simulink model "test_phase_voltages_without_delays"  (R2022a)
settings: Solver=FixedStepDiscrete  StartTime=0.0  StopTime=10.0  RelTol=1e-3
undefined symbols (not defined in the file or in its folder): f_c, Rt, u_dc
libraries: hdlsllib x3, simulink x2
(part 1 of 2)
settings Model: DataTypeOverride=Off  Creator=Andre Merx  LastModifiedBy=Andre Merx
settings SolverCC: AlgebraicLoopSolver=TrustRegion
settings DataIOCC: LimitDataPoints=on  SaveOutput=off  SaveTime=off
settings OptimizationCC: BlockReduction=off  ConditionallyExecuteInputs=off  DefaultParameterBehavior=Inlined  LifeSpan=inf
settings DebuggingCC: AlgebraicLoopMsg=error  SingleTaskRateTransMsg=error  UnconnectedInputMsg=warning  UnconnectedOutputMsg=warning  UnconnectedLineMsg=warning  AllowSymbolicDim=off  StrictBusMsg=ErrorOnBusTreatedAsVector  SFUnexpectedBacktrackingDiag=warning  SFNoUnconditionalDefaultTransitionDiag=warning  SFExecutionAtInitializationDiag=none  SFMachineParentedDataDiag=warning  ArithmeticOperatorsInVariantConditions=warning
settings HardwareCC: ProdBitPerPointer=32  ProdBitPerSizeT=32  ProdBitPerPtrDiffT=32  ProdLargestAtomicFloat=None  ProdIntDivRoundTo=Undefined  ProdEndianess=Unspecified  ProdWordSize=32  ProdHWDeviceType=ASIC/FPGA->ASIC/FPGA  ProdEqTarget=off
settings SFSimCC: SimUseLocalCustomCode=off  CustomCodeUndefinedFunction=UseInterfaceOnly
settings RTWCC: RTWUseLocalCustomCode=off
settings CodeAppCC: StateflowObjectComments=on
settings GRTTargetCC: TargetLangStandard=C89/C90 (ANSI)
settings ConfigComp: CovScope=ReferencedModels  CovMetricSettings=dw  CovSaveCumulativeToWorkspaceVar=on  CovSaveSingleToWorkspaceVar=on  CovExternalEMLEnable=off  CovSFcnEnable=off

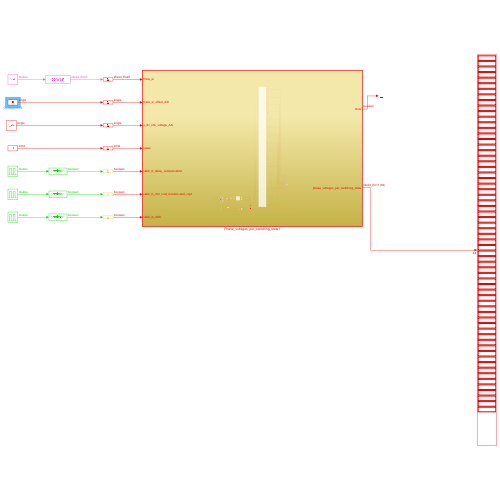
[thumbnail: Simulink's stored preview of the top-level diagram]
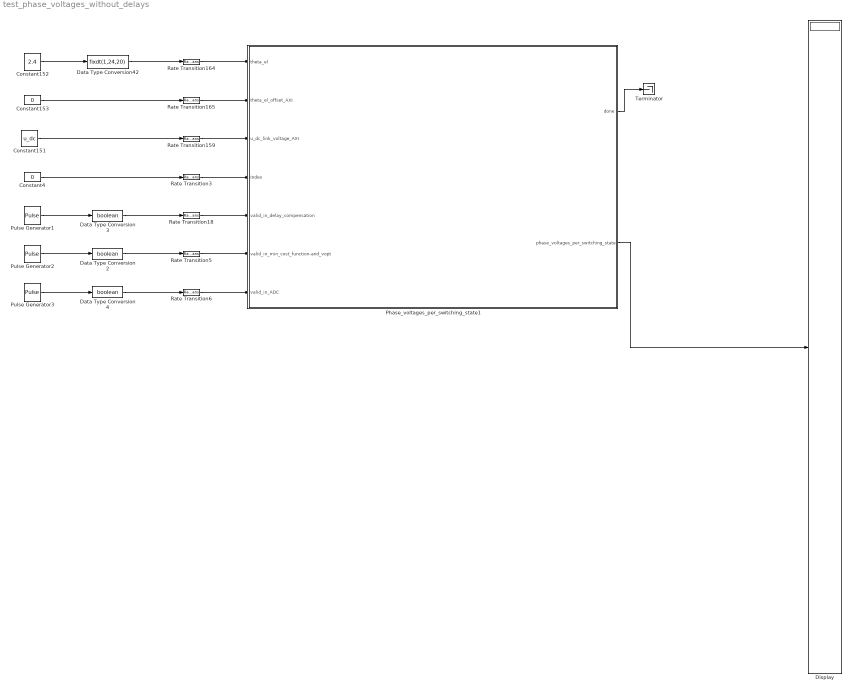
== system test_phase_voltages_without_delays ==
  Constant151 : Constant  Value=u_dc  OutDataTypeStr=single  SampleTime=-1
  Constant152 : Constant  Value=2.4
  Constant153 : Constant  Value=0  OutDataTypeStr=fixdt(1,24,20)  SampleTime=-1
  Constant4 : Constant  Value=0  OutDataTypeStr=int32  SampleTime=-1
  Data Type Conversion2 : DataTypeConversion  OutDataTypeStr=boolean  SaturateOnIntegerOverflow=off  RndMeth=Floor
  Data Type Conversion3 : DataTypeConversion  OutDataTypeStr=boolean  SaturateOnIntegerOverflow=off  RndMeth=Floor
  Data Type Conversion4 : DataTypeConversion  OutDataTypeStr=boolean  SaturateOnIntegerOverflow=off  RndMeth=Floor
  Data Type Conversion42 : DataTypeConversion  OutDataTypeStr=fixdt(1,24,20)  SaturateOnIntegerOverflow=off  RndMeth=Floor
  Display : Display
  Phase_voltages_per_switching_state1 : Subsystem  TreatAsAtomicUnit=on
  Pulse Generator1 : DiscretePulseGenerator  PulseType=Time based  Period=1/f_c
  Pulse Generator2 : DiscretePulseGenerator  PulseType=Time based  Period=1/f_c
  Pulse Generator3 : DiscretePulseGenerator  PulseType=Time based  Period=1/f_c
  Rate Transition{3,5..6,18,159,164..165} (7 alike) : RateTransition  OutPortSampleTime=Rt
  Terminator : Terminator
  wires:
  Rate Transition165/1 -> Phase_voltages_per_switching_state1/2(theta_el_offset_AXI)
  Rate Transition164/1 -> Phase_voltages_per_switching_state1/1(theta_el)
  Rate Transition159/1 -> Phase_voltages_per_switching_state1/3(u_dc_link_voltage_AXI)
  Constant152/1 -> Data Type Conversion42/1
  Constant153/1 -> Rate Transition165/1
  Constant151/1 -> Rate Transition159/1
  Data Type Conversion42/1 -> Rate Transition164/1
  Data Type Conversion3/1 -> Rate Transition18/1
  Rate Transition6/1 -> Phase_voltages_per_switching_state1/7(valid_in_ADC)
  Rate Transition18/1 -> Phase_voltages_per_switching_state1/5(valid_in_delay_compensation)
  Pulse Generator1/1 -> Data Type Conversion3/1
  Rate Transition3/1 -> Phase_voltages_per_switching_state1/4(Index)
  Data Type Conversion4/1 -> Rate Transition6/1
  Constant4/1 -> Rate Transition3/1
  Data Type Conversion2/1 -> Rate Transition5/1
  Pulse Generator3/1 -> Data Type Conversion4/1
  Rate Transition5/1 -> Phase_voltages_per_switching_state1/6(valid_in_min_cost_function-and_vopt)
  Pulse Generator2/1 -> Data Type Conversion2/1
  Phase_voltages_per_switching_state1/1(done) -> Terminator/1
  Phase_voltages_per_switching_state1/2(phase_voltages_per_switching_state) -> Display/1

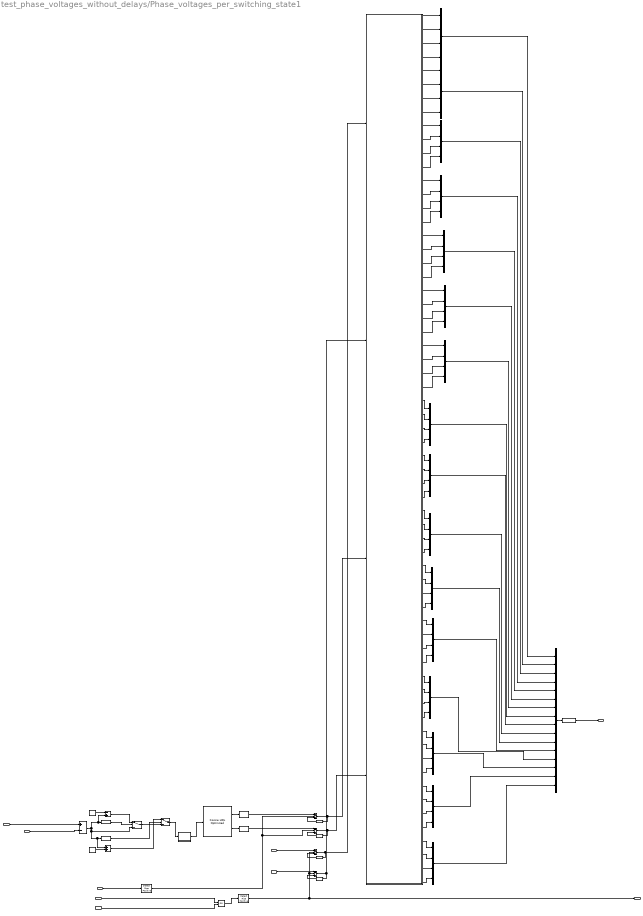
== system test_phase_voltages_without_delays/Phase_voltages_per_switching_state1 ==
  theta_el : Inport
  theta_el_offset_AXI : Inport  Port=2
  u_dc_link_voltage_AXI : Inport  Port=3
  Index : Inport  Port=4
  valid_in_delay_compensation : Inport  Port=5
  valid_in_min_cost_function-and_vopt : Inport  Port=6
  valid_in_ADC : Inport  Port=7
  Add1 : Sum  Inputs=+-  OutDataTypeStr=fixdt(1,24,20)
  Add2 : Sum  Inputs=-+  OutDataTypeStr=fixdt(1,24,20)
  Add3 : Sum  OutDataTypeStr=fixdt(1,24,20)
  Compare Limit_High : simulink/Logic and Bit Operations/Compare To Constant  relop=>=  const=2*pi  OutDataTypeStr=boolean
  Compare Limit_Low : simulink/Logic and Bit Operations/Compare To Constant  relop=<  const=0  OutDataTypeStr=boolean
  Constant : Constant  Value=2*pi  OutDataTypeStr=fixdt(1,24,20)  SampleTime=Rt
  Constant1 : Constant  Value=2*pi  OutDataTypeStr=fixdt(1,24,20)  SampleTime=Rt
  Data Type Conversion1 : DataTypeConversion  OutDataTypeStr=fixdt(1,24,11)  SaturateOnIntegerOverflow=off  RndMeth=Floor
  Data Type Conversion2 : DataTypeConversion  OutDataTypeStr=single  SaturateOnIntegerOverflow=off  RndMeth=Floor
  Data Type Conversion42 : DataTypeConversion  OutDataTypeStr=single  SaturateOnIntegerOverflow=off  RndMeth=Floor
  Delay{1..2,13..14} (4 alike) : Delay  DelayLength=1
  Detect Rise Positive : hdlsllib/Logic and Bit Operations/Detect Rise Positive  vinit=0  OutDataTypeStr=boolean
      settings: SourceProductBaseCode=SL
  Detect Rise Positive1 : hdlsllib/Logic and Bit Operations/Detect Rise Positive  vinit=0  OutDataTypeStr=boolean
      settings: SourceProductBaseCode=SL
  Logical Operator : Logic  Operator=OR  AllPortsSameDT=off  OutDataTypeStr=boolean
  MATLAB Function1 : MATLAB Function  TreatAsAtomicUnit=on
  Mux{,1..15} (16 alike) : Mux
  Mux16 : Mux  Inputs=16
  Sine HDL Optimized : hdlsllib/Lookup Tables/Cosine HDL Optimized  OutputFormula=sin(2*pi*u) and cos(2*pi*u)  NumDataPoints=64  TableDataTypeStr=fixdt(1,24,20)  SimulateLUTROMDelay=off
      settings: SourceProductBaseCode=SL
  Subsystem : Subsystem
  Switch_Limit_High : Switch  Criteria=u2 > Threshold  OutDataTypeStr=fixdt(1,24,20)  SaturateOnIntegerOverflow=off  InputSameDT=off
  Switch_Limit_Low : Switch  Criteria=u2 > Threshold  OutDataTypeStr=fixdt(1,24,20)  SaturateOnIntegerOverflow=off  InputSameDT=off
  Switch_on1 : Switch  Threshold=1  OutDataTypeStr=single  RndMeth=Simplest  SaturateOnIntegerOverflow=off  InputSameDT=off
  Switch_on13 : Switch  Threshold=1  OutDataTypeStr=single  RndMeth=Simplest  SaturateOnIntegerOverflow=off  InputSameDT=off
  Switch_on2 : Switch  Threshold=1  OutDataTypeStr=single  RndMeth=Simplest  SaturateOnIntegerOverflow=off  InputSameDT=off
  Switch_on3 : Switch  Threshold=1  OutDataTypeStr=int32  RndMeth=Simplest  SaturateOnIntegerOverflow=off  InputSameDT=off
  done : Outport
  phase_voltages_per_switching_state : Outport  Port=2
  wires:
  Compare Limit_High/1 -> Switch_Limit_High/2
  Delay14/1 -> Switch_on3/3
  Delay13/1 -> Switch_on13/3
  Switch_on13/1 -> Subsystem/4(cos_theta_el1), Delay13/1
  u_dc_link_voltage_AXI/1 -> Switch_on1/1  "End_Cycle"
  Switch_Limit_High/1 -> Switch_Limit_Low/3
  Constant/1 -> Add2/1
  theta_el_offset_AXI/1 -> Add1/2
  Add3/1 -> Switch_Limit_Low/1
  theta_el/1 -> Add1/1  "End_Cycle"
  Switch_Limit_Low/1 -> MATLAB Function1/1(u)  "End_Cycle"
  Add1/1 -> Switch_Limit_High/3, Add3/1, Compare Limit_Low/1, Add2/2, Compare Limit_High/1
  Switch_on1/1 -> Subsystem/1(u_dc_link_voltage15), Delay1/1
  Detect Rise Positive1/1 -> done/1, Switch_on3/2, Switch_on1/2  "End_Cycle"
  Compare Limit_Low/1 -> Switch_Limit_Low/2
  Delay1/1 -> Switch_on1/3
  Constant1/1 -> Add3/2
  Add2/1 -> Switch_Limit_High/1
  Index/1 -> Switch_on3/1  "End_Cycle"
  Logical Operator/1 -> Detect Rise Positive1/1
  Switch_on3/1 -> Delay14/1, Subsystem/2(Index 15)
  Subsystem/61(d_voltage_per_switching_state15) -> Mux/1
  Subsystem/62(q_voltage_per_switching_state15) -> Mux/2
  Subsystem/63(x_voltage_per_switching_state15) -> Mux/3
  Subsystem/64(y_voltage_per_switching_state15) -> Mux/4
  Subsystem/1(d_voltage_per_switching_state) -> Mux1/1
  Subsystem/2(q_voltage_per_switching_state) -> Mux1/2
  Subsystem/4(y_voltage_per_switching_state) -> Mux1/4
  Subsystem/3(x_voltage_per_switching_state) -> Mux1/3
  Subsystem/7(x_voltage_per_switching_state1) -> Mux2/3
  Subsystem/5(d_voltage_per_switching_state1) -> Mux2/1
  Subsystem/6(q_voltage_per_switching_state1) -> Mux2/2
  Subsystem/8(y_voltage_per_switching_state1) -> Mux2/4
  Subsystem/12(y_voltage_per_switching_state2) -> Mux3/4
  Subsystem/9(d_voltage_per_switching_state2) -> Mux3/1
  Subsystem/10(q_voltage_per_switching_state2) -> Mux3/2
  Subsystem/11(x_voltage_per_switching_state2) -> Mux3/3
  Subsystem/13(d_voltage_per_switching_state3) -> Mux4/1
  Subsystem/15(x_voltage_per_switching_state3) -> Mux4/3
  Subsystem/16(y_voltage_per_switching_state3) -> Mux4/4
  Subsystem/14(q_voltage_per_switching_state3) -> Mux4/2
  Subsystem/19(x_voltage_per_switching_state4) -> Mux5/3
  Subsystem/18(q_voltage_per_switching_state4) -> Mux5/2
  Subsystem/17(d_voltage_per_switching_state4) -> Mux5/1
  Subsystem/20(y_voltage_per_switching_state4) -> Mux5/4
  Subsystem/23(x_voltage_per_switching_state5) -> Mux6/3
  Subsystem/21(d_voltage_per_switching_state5) -> Mux6/1
  Subsystem/22(q_voltage_per_switching_state5) -> Mux6/2
  Subsystem/24(y_voltage_per_switching_state5) -> Mux6/4
  Subsystem/25(d_voltage_per_switching_state6) -> Mux7/1
  Subsystem/28(y_voltage_per_switching_state6) -> Mux7/4
  Subsystem/27(x_voltage_per_switching_state6) -> Mux7/3
  Subsystem/26(q_voltage_per_switching_state6) -> Mux7/2
  Subsystem/29(d_voltage_per_switching_state7) -> Mux8/1
  Subsystem/32(y_voltage_per_switching_state7) -> Mux8/4
  Subsystem/30(q_voltage_per_switching_state7) -> Mux8/2
  Subsystem/31(x_voltage_per_switching_state7) -> Mux8/3
  Subsystem/36(y_voltage_per_switching_state8) -> Mux9/4
  Subsystem/33(d_voltage_per_switching_state8) -> Mux9/1
  Subsystem/34(q_voltage_per_switching_state8) -> Mux9/2
  Subsystem/35(x_voltage_per_switching_state8) -> Mux9/3
  Mux10/1 -> Mux16/10
  Subsystem/40(y_voltage_per_switching_state9) -> Mux10/4
  Subsystem/39(x_voltage_per_switching_state9) -> Mux10/3
  Subsystem/37(d_voltage_per_switching_state9) -> Mux10/1
  Subsystem/38(q_voltage_per_switching_state9) -> Mux10/2
  Subsystem/43(x_voltage_per_switching_state10) -> Mux11/3
  Subsystem/41(d_voltage_per_switching_state10) -> Mux11/1
  Subsystem/42(q_voltage_per_switching_state10) -> Mux11/2
  Subsystem/44(y_voltage_per_switching_state10) -> Mux11/4
  Mux12/1 -> Mux16/12
  Subsystem/48(y_voltage_per_switching_state11) -> Mux12/4
  Subsystem/46(q_voltage_per_switching_state11) -> Mux12/2
  Subsystem/47(x_voltage_per_switching_state11) -> Mux12/3
  Subsystem/45(d_voltage_per_switching_state11) -> Mux12/1
  Subsystem/52(y_voltage_per_switching_state12) -> Mux13/4
  Subsystem/50(q_voltage_per_switching_state12) -> Mux13/2
  Subsystem/51(x_voltage_per_switching_state12) -> Mux13/3
  Subsystem/49(d_voltage_per_switching_state12) -> Mux13/1
  Mux14/1 -> Mux16/14
  Subsystem/56(y_voltage_per_switching_state13) -> Mux14/4
  Subsystem/53(d_voltage_per_switching_state13) -> Mux14/1
  Subsystem/55(x_voltage_per_switching_state13) -> Mux14/3
  Subsystem/54(q_voltage_per_switching_state13) -> Mux14/2
  Subsystem/57(d_voltage_per_switching_state14) -> Mux15/1
  Subsystem/60(y_voltage_per_switching_state14) -> Mux15/4
  Subsystem/59(x_voltage_per_switching_state14) -> Mux15/3
  Subsystem/58(q_voltage_per_switching_state14) -> Mux15/2
  Mux15/1 -> Mux16/15
  Mux16/1 -> Data Type Conversion1/1
  Mux1/1 -> Mux16/1
  Mux2/1 -> Mux16/2
  Mux3/1 -> Mux16/3
  Mux4/1 -> Mux16/4
  Mux5/1 -> Mux16/5
  Mux6/1 -> Mux16/6
  Mux7/1 -> Mux16/7
  Mux8/1 -> Mux16/8
  Mux9/1 -> Mux16/9
  Mux11/1 -> Mux16/11
  Mux13/1 -> Mux16/13
  Mux/1 -> Mux16/16
  Data Type Conversion1/1 -> phase_voltages_per_switching_state/1
  valid_in_ADC/1 -> Detect Rise Positive/1
  valid_in_delay_compensation/1 -> Logical Operator/1
  valid_in_min_cost_function-and_vopt/1 -> Logical Operator/2
  MATLAB Function1/1(y) -> Sine HDL Optimized/1
  Sine HDL Optimized/1 -> Data Type Conversion42/1
  Detect Rise Positive/1 -> Switch_on13/2, Switch_on2/2  "End_Cycle"
  Delay2/1 -> Switch_on2/3
  Switch_on2/1 -> Subsystem/3(sin_theta_el), Delay2/1
  Sine HDL Optimized/2 -> Data Type Conversion2/1
  Data Type Conversion42/1 -> Switch_on2/1
  Data Type Conversion2/1 -> Switch_on13/1

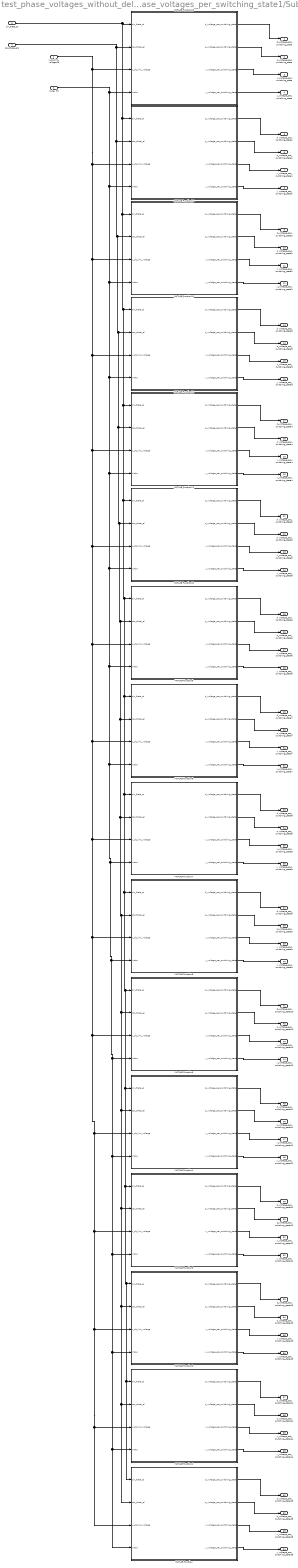
== system test_phase_voltages_without_delays/Phase_voltages_per_switching_state1/Subsystem ==
  u_dc_link_voltage15 : Inport
  Index 15 : Inport  Port=2
  sin_theta_el : Inport  Port=3
  cos_theta_el1 : Inport  Port=4
  MATLAB Function : MATLAB Function  TreatAsAtomicUnit=on
  MATLAB Function1 : MATLAB Function  TreatAsAtomicUnit=on
  MATLAB Function10 : MATLAB Function  TreatAsAtomicUnit=on
  MATLAB Function11 : MATLAB Function  TreatAsAtomicUnit=on
  MATLAB Function12 : MATLAB Function  TreatAsAtomicUnit=on
  MATLAB Function13 : MATLAB Function  TreatAsAtomicUnit=on
  MATLAB Function14 : MATLAB Function  TreatAsAtomicUnit=on
  MATLAB Function15 : MATLAB Function  TreatAsAtomicUnit=on
  MATLAB Function2 : MATLAB Function  TreatAsAtomicUnit=on
  MATLAB Function3 : MATLAB Function  TreatAsAtomicUnit=on
  MATLAB Function4 : MATLAB Function  TreatAsAtomicUnit=on
  MATLAB Function5 : MATLAB Function  TreatAsAtomicUnit=on
  MATLAB Function6 : MATLAB Function  TreatAsAtomicUnit=on
  MATLAB Function7 : MATLAB Function  TreatAsAtomicUnit=on
  MATLAB Function8 : MATLAB Function  TreatAsAtomicUnit=on
  MATLAB Function9 : MATLAB Function  TreatAsAtomicUnit=on
  d_voltage_per_switching_state : Outport
  q_voltage_per_switching_state : Outport  Port=2
  x_voltage_per_switching_state : Outport  Port=3
  y_voltage_per_switching_state : Outport  Port=4
  d_voltage_per_switching_state1 : Outport  Port=5
  q_voltage_per_switching_state1 : Outport  Port=6
  x_voltage_per_switching_state1 : Outport  Port=7
  y_voltage_per_switching_state1 : Outport  Port=8
  d_voltage_per_switching_state2 : Outport  Port=9
  q_voltage_per_switching_state2 : Outport  Port=10
  x_voltage_per_switching_state2 : Outport  Port=11
  y_voltage_per_switching_state2 : Outport  Port=12
  d_voltage_per_switching_state3 : Outport  Port=13
  q_voltage_per_switching_state3 : Outport  Port=14
  x_voltage_per_switching_state3 : Outport  Port=15
  y_voltage_per_switching_state3 : Outport  Port=16
  d_voltage_per_switching_state4 : Outport  Port=17
  q_voltage_per_switching_state4 : Outport  Port=18
  x_voltage_per_switching_state4 : Outport  Port=19
  y_voltage_per_switching_state4 : Outport  Port=20
  d_voltage_per_switching_state5 : Outport  Port=21
  q_voltage_per_switching_state5 : Outport  Port=22
  x_voltage_per_switching_state5 : Outport  Port=23
  y_voltage_per_switching_state5 : Outport  Port=24
  d_voltage_per_switching_state6 : Outport  Port=25
  q_voltage_per_switching_state6 : Outport  Port=26
  x_voltage_per_switching_state6 : Outport  Port=27
  y_voltage_per_switching_state6 : Outport  Port=28
  d_voltage_per_switching_state7 : Outport  Port=29
  q_voltage_per_switching_state7 : Outport  Port=30
  x_voltage_per_switching_state7 : Outport  Port=31
  y_voltage_per_switching_state7 : Outport  Port=32
  d_voltage_per_switching_state8 : Outport  Port=33
  q_voltage_per_switching_state8 : Outport  Port=34
  x_voltage_per_switching_state8 : Outport  Port=35
  y_voltage_per_switching_state8 : Outport  Port=36
  d_voltage_per_switching_state9 : Outport  Port=37
  q_voltage_per_switching_state9 : Outport  Port=38
  x_voltage_per_switching_state9 : Outport  Port=39
  y_voltage_per_switching_state9 : Outport  Port=40
  d_voltage_per_switching_state10 : Outport  Port=41
  q_voltage_per_switching_state10 : Outport  Port=42
  x_voltage_per_switching_state10 : Outport  Port=43
  y_voltage_per_switching_state10 : Outport  Port=44
  d_voltage_per_switching_state11 : Outport  Port=45
  q_voltage_per_switching_state11 : Outport  Port=46
  x_voltage_per_switching_state11 : Outport  Port=47
  y_voltage_per_switching_state11 : Outport  Port=48
  d_voltage_per_switching_state12 : Outport  Port=49
  q_voltage_per_switching_state12 : Outport  Port=50
  x_voltage_per_switching_state12 : Outport  Port=51
  y_voltage_per_switching_state12 : Outport  Port=52
  d_voltage_per_switching_state13 : Outport  Port=53
  q_voltage_per_switching_state13 : Outport  Port=54
  x_voltage_per_switching_state13 : Outport  Port=55
  y_voltage_per_switching_state13 : Outport  Port=56
  d_voltage_per_switching_state14 : Outport  Port=57
  q_voltage_per_switching_state14 : Outport  Port=58
  x_voltage_per_switching_state14 : Outport  Port=59
  y_voltage_per_switching_state14 : Outport  Port=60
  d_voltage_per_switching_state15 : Outport  Port=61
  q_voltage_per_switching_state15 : Outport  Port=62
  x_voltage_per_switching_state15 : Outport  Port=63
  y_voltage_per_switching_state15 : Outport  Port=64
  wires:
  MATLAB Function4/1(d_voltage_per_switching_state) -> d_voltage_per_switching_state11/1
  MATLAB Function11/4(y_voltage_per_switching_state) -> y_voltage_per_switching_state4/1
  MATLAB Function3/2(q_voltage_per_switching_state) -> q_voltage_per_switching_state12/1
  MATLAB Function3/4(y_voltage_per_switching_state) -> y_voltage_per_switching_state12/1
  MATLAB Function10/3(x_voltage_per_switching_state) -> x_voltage_per_switching_state5/1
  MATLAB Function8/1(d_voltage_per_switching_state) -> d_voltage_per_switching_state7/1
  MATLAB Function8/2(q_voltage_per_switching_state) -> q_voltage_per_switching_state7/1
  MATLAB Function3/1(d_voltage_per_switching_state) -> d_voltage_per_switching_state12/1
  MATLAB Function11/1(d_voltage_per_switching_state) -> d_voltage_per_switching_state4/1
  MATLAB Function12/3(x_voltage_per_switching_state) -> x_voltage_per_switching_state3/1
  MATLAB Function15/2(q_voltage_per_switching_state) -> q_voltage_per_switching_state/1
  MATLAB Function8/3(x_voltage_per_switching_state) -> x_voltage_per_switching_state7/1
  MATLAB Function/1(d_voltage_per_switching_state) -> d_voltage_per_switching_state15/1
  MATLAB Function11/3(x_voltage_per_switching_state) -> x_voltage_per_switching_state4/1
  MATLAB Function10/4(y_voltage_per_switching_state) -> y_voltage_per_switching_state5/1
  MATLAB Function4/3(x_voltage_per_switching_state) -> x_voltage_per_switching_state11/1
  MATLAB Function11/2(q_voltage_per_switching_state) -> q_voltage_per_switching_state4/1
  MATLAB Function12/1(d_voltage_per_switching_state) -> d_voltage_per_switching_state3/1
  MATLAB Function2/1(d_voltage_per_switching_state) -> d_voltage_per_switching_state13/1
  MATLAB Function12/4(y_voltage_per_switching_state) -> y_voltage_per_switching_state3/1
  MATLAB Function/3(x_voltage_per_switching_state) -> x_voltage_per_switching_state15/1
  MATLAB Function13/2(q_voltage_per_switching_state) -> q_voltage_per_switching_state2/1
  MATLAB Function10/1(d_voltage_per_switching_state) -> d_voltage_per_switching_state5/1
  MATLAB Function10/2(q_voltage_per_switching_state) -> q_voltage_per_switching_state5/1
  MATLAB Function4/4(y_voltage_per_switching_state) -> y_voltage_per_switching_state11/1
  MATLAB Function3/3(x_voltage_per_switching_state) -> x_voltage_per_switching_state12/1
  MATLAB Function13/4(y_voltage_per_switching_state) -> y_voltage_per_switching_state2/1
  MATLAB Function8/4(y_voltage_per_switching_state) -> y_voltage_per_switching_state7/1
  MATLAB Function13/1(d_voltage_per_switching_state) -> d_voltage_per_switching_state2/1
  MATLAB Function13/3(x_voltage_per_switching_state) -> x_voltage_per_switching_state2/1
  MATLAB Function1/4(y_voltage_per_switching_state) -> y_voltage_per_switching_state14/1
  MATLAB Function1/1(d_voltage_per_switching_state) -> d_voltage_per_switching_state14/1
  MATLAB Function12/2(q_voltage_per_switching_state) -> q_voltage_per_switching_state3/1
  MATLAB Function4/2(q_voltage_per_switching_state) -> q_voltage_per_switching_state11/1
  MATLAB Function6/2(q_voltage_per_switching_state) -> q_voltage_per_switching_state9/1
  MATLAB Function5/3(x_voltage_per_switching_state) -> x_voltage_per_switching_state10/1
  MATLAB Function6/3(x_voltage_per_switching_state) -> x_voltage_per_switching_state9/1
  MATLAB Function6/1(d_voltage_per_switching_state) -> d_voltage_per_switching_state9/1
  MATLAB Function6/4(y_voltage_per_switching_state) -> y_voltage_per_switching_state9/1
  MATLAB Function15/1(d_voltage_per_switching_state) -> d_voltage_per_switching_state/1
  MATLAB Function15/4(y_voltage_per_switching_state) -> y_voltage_per_switching_state/1
  MATLAB Function15/3(x_voltage_per_switching_state) -> x_voltage_per_switching_state/1
  MATLAB Function/4(y_voltage_per_switching_state) -> y_voltage_per_switching_state15/1
  MATLAB Function/2(q_voltage_per_switching_state) -> q_voltage_per_switching_state15/1
  u_dc_link_voltage15/1 -> MATLAB Function/3(u_dc_link_voltage), MATLAB Function1/3(u_dc_link_voltage), MATLAB Function2/3(u_dc_link_voltage), MATLAB Function3/3(u_dc_link_voltage), MATLAB Function4/3(u_dc_link_voltage), MATLAB Function5/3(u_dc_link_voltage), MATLAB Function6/3(u_dc_link_voltage), MATLAB Function7/3(u_dc_link_voltage), MATLAB Function8/3(u_dc_link_voltage), MATLAB Function9/3(u_dc_link_voltage), MATLAB Function10/3(u_dc_link_voltage), MATLAB Function11/3(u_dc_link_voltage), MATLAB Function12/3(u_dc_link_voltage), MATLAB Function13/3(u_dc_link_voltage), MATLAB Function14/3(u_dc_link_voltage), MATLAB Function15/3(u_dc_link_voltage)
  MATLAB Function14/4(y_voltage_per_switching_state) -> y_voltage_per_switching_state1/1
  MATLAB Function2/2(q_voltage_per_switching_state) -> q_voltage_per_switching_state13/1
  MATLAB Function14/3(x_voltage_per_switching_state) -> x_voltage_per_switching_state1/1
  MATLAB Function14/1(d_voltage_per_switching_state) -> d_voltage_per_switching_state1/1
  MATLAB Function14/2(q_voltage_per_switching_state) -> q_voltage_per_switching_state1/1
  Index 15/1 -> MATLAB Function15/4(Index), MATLAB Function10/4(Index), MATLAB Function8/4(Index), MATLAB Function/4(Index), MATLAB Function1/4(Index), MATLAB Function2/4(Index), MATLAB Function3/4(Index), MATLAB Function4/4(Index), MATLAB Function5/4(Index), MATLAB Function6/4(Index), MATLAB Function7/4(Index), MATLAB Function9/4(Index), MATLAB Function11/4(Index), MATLAB Function12/4(Index), MATLAB Function13/4(Index), MATLAB Function14/4(Index)
  MATLAB Function1/2(q_voltage_per_switching_state) -> q_voltage_per_switching_state14/1
  MATLAB Function1/3(x_voltage_per_switching_state) -> x_voltage_per_switching_state14/1
  MATLAB Function9/3(x_voltage_per_switching_state) -> x_voltage_per_switching_state6/1
  MATLAB Function9/2(q_voltage_per_switching_state) -> q_voltage_per_switching_state6/1
  MATLAB Function9/1(d_voltage_per_switching_state) -> d_voltage_per_switching_state6/1
  MATLAB Function9/4(y_voltage_per_switching_state) -> y_voltage_per_switching_state6/1
  MATLAB Function7/1(d_voltage_per_switching_state) -> d_voltage_per_switching_state8/1
  MATLAB Function7/4(y_voltage_per_switching_state) -> y_voltage_per_switching_state8/1
  MATLAB Function7/2(q_voltage_per_switching_state) -> q_voltage_per_switching_state8/1
  MATLAB Function7/3(x_voltage_per_switching_state) -> x_voltage_per_switching_state8/1
  MATLAB Function5/2(q_voltage_per_switching_state) -> q_voltage_per_switching_state10/1
  MATLAB Function5/1(d_voltage_per_switching_state) -> d_voltage_per_switching_state10/1
  MATLAB Function5/4(y_voltage_per_switching_state) -> y_voltage_per_switching_state10/1
  MATLAB Function2/3(x_voltage_per_switching_state) -> x_voltage_per_switching_state13/1
  MATLAB Function2/4(y_voltage_per_switching_state) -> y_voltage_per_switching_state13/1
  sin_theta_el/1 -> MATLAB Function14/1(sin_theta_el), MATLAB Function/1(sin_theta_el), MATLAB Function1/1(sin_theta_el), MATLAB Function2/1(sin_theta_el), MATLAB Function3/1(sin_theta_el), MATLAB Function4/1(sin_theta_el), MATLAB Function5/1(sin_theta_el), MATLAB Function6/1(sin_theta_el), MATLAB Function7/1(sin_theta_el), MATLAB Function8/1(sin_theta_el), MATLAB Function9/1(sin_theta_el), MATLAB Function10/1(sin_theta_el), MATLAB Function11/1(sin_theta_el), MATLAB Function12/1(sin_theta_el), MATLAB Function13/1(sin_theta_el), MATLAB Function15/1(sin_theta_el)
  cos_theta_el1/1 -> MATLAB Function15/2(cos_theta_el), MATLAB Function/2(cos_theta_el), MATLAB Function1/2(cos_theta_el), MATLAB Function2/2(cos_theta_el), MATLAB Function3/2(cos_theta_el), MATLAB Function4/2(cos_theta_el), MATLAB Function5/2(cos_theta_el), MATLAB Function6/2(cos_theta_el), MATLAB Function7/2(cos_theta_el), MATLAB Function8/2(cos_theta_el), MATLAB Function9/2(cos_theta_el), MATLAB Function10/2(cos_theta_el), MATLAB Function11/2(cos_theta_el), MATLAB Function12/2(cos_theta_el), MATLAB Function13/2(cos_theta_el), MATLAB Function14/2(cos_theta_el)

== matlab function test_phase_voltages_without_delays/Phase_voltages_per_switching_state1/Subsystem/MATLAB Function14 ==
  data: sin_theta_el input; cos_theta_el input; d_voltage_per_switching_state output; u_dc_link_voltage input; Index input; q_voltage_per_switching_state output; x_voltage_per_switching_state output; y_voltage_per_switching_state output
function [d_voltage_per_switching_state, q_voltage_per_switching_state, x_voltage_per_switching_state, y_voltage_per_switching_state] = fcn(sin_theta_el, cos_theta_el, u_dc_link_voltage, Index)
      
        % Initial condition
            Index = Index+1;

    
        % Swichtingstates factors alpha beta x y
        Factors_alpha_beta_x_y = single([-0.166666666666667	 0.166666666666667	-0.333333333333333	0;
                                         -0.288675134594813	-0.288675134594813	 0	                0;
                                         -0.166666666666667	 0.166666666666667	-0.333333333333333	0;
                                          0.288675134594813	 0.288675134594813	 0              	0]);
        
        % Park-Transformation of the switchingstates factors
        Factors_d_q_x_y =single(zeros(4,1));
    
        Factors_d_q_x_y(3,1) = Factors_alpha_beta_x_y(3,Index);
        Factors_d_q_x_y(4,1) = Factors_alpha_beta_x_y(4,Index);
       
        Factors_d_q_x_y(1,1) = cos_theta_el*Factors_alpha_beta_x_y(1,Index)+sin_theta_el*Factors_alpha_beta_x_y(2,Index);
        Factors_d_q_x_y(2,1) = -sin_theta_el*Factors_alpha_beta_x_y(1,Index)+cos_theta_el*Factors_alpha_beta_x_y(2,Index);
    
        %Calculation of the voltages per switching state in alpha beta coordinates
        d_q_x_y_voltages_per_switching_state = single(u_dc_link_voltage*Factors_d_q_x_y);
    
        d_voltage_per_switching_state = d_q_x_y_voltages_per_switching_state(1,1);
        q_voltage_per_switching_state = d_q_x_y_voltages_per_switching_state(2,1);
        x_voltage_per_switching_state = d_q_x_y_voltages_per_switching_state(3,1);
        y_voltage_per_switching_state = d_q_x_y_voltages_per_switching_state(4,1);
    

end

== matlab function test_phase_voltages_without_delays/Phase_voltages_per_switching_state1/Subsystem/MATLAB Function15 ==
  data: sin_theta_el input; cos_theta_el input; d_voltage_per_switching_state output; u_dc_link_voltage input; Index input; q_voltage_per_switching_state output; x_voltage_per_switching_state output; y_voltage_per_switching_state output
function [d_voltage_per_switching_state, q_voltage_per_switching_state, x_voltage_per_switching_state, y_voltage_per_switching_state] = fcn(sin_theta_el, cos_theta_el, u_dc_link_voltage, Index)
      
        % Initial condition
            Index = Index+1;

        % Swichtingstates factors alpha beta x y
        Factors_alpha_beta_x_y = single([0	    0.333333333333333	-0.166666666666667	 0.166666666666667;
                                         0	    0                    0.288675134594813	 0.288675134594813;
                                         0	    0.333333333333333	-0.166666666666667	 0.166666666666667;
                                         0	    0	                -0.288675134594813	-0.288675134594813]);
        
        % Park-Transformation of the switchingstates factors
        Factors_d_q_x_y =single(zeros(4,1));
    
        Factors_d_q_x_y(3,1) = Factors_alpha_beta_x_y(3,Index);
        Factors_d_q_x_y(4,1) = Factors_alpha_beta_x_y(4,Index);
          
        Factors_d_q_x_y(1,1) = cos_theta_el*Factors_alpha_beta_x_y(1,Index)+sin_theta_el*Factors_alpha_beta_x_y(2,Index);
        Factors_d_q_x_y(2,1) = -sin_theta_el*Factors_alpha_beta_x_y(1,Index)+cos_theta_el*Factors_alpha_beta_x_y(2,Index);
    
        %Calculation of the voltages per switching state in alpha beta coordinates
        d_q_x_y_voltages_per_switching_state = single(u_dc_link_voltage*Factors_d_q_x_y);
    
        d_voltage_per_switching_state = d_q_x_y_voltages_per_switching_state(1,1);
        q_voltage_per_switching_state = d_q_x_y_voltages_per_switching_state(2,1);
        x_voltage_per_switching_state = d_q_x_y_voltages_per_switching_state(3,1);
        y_voltage_per_switching_state = d_q_x_y_voltages_per_switching_state(4,1);
    

end

== matlab function test_phase_voltages_without_delays/Phase_voltages_per_switching_state1/Subsystem/MATLAB Function2 ==
  data: sin_theta_el input; cos_theta_el input; d_voltage_per_switching_state output; u_dc_link_voltage input; Index input; q_voltage_per_switching_state output; x_voltage_per_switching_state output; y_voltage_per_switching_state output
function [d_voltage_per_switching_state, q_voltage_per_switching_state, x_voltage_per_switching_state, y_voltage_per_switching_state] = fcn(sin_theta_el, cos_theta_el, u_dc_link_voltage, Index)
      
        % Initial condition
            Index = Index+1;

        % Swichtingstates factors alpha beta x y
        Factors_alpha_beta_x_y = single([-0.455341801261480	-0.122008467928146	-0.622008467928146	-0.288675134594813;
                                         -0.455341801261480	-0.455341801261480	-0.166666666666667	-0.166666666666667;
                                         0.122008467928146	 0.455341801261480	-0.0446581987385205  0.288675134594813;
                                         0.122008467928146	 0.122008467928146	-0.166666666666667	-0.166666666666667]);
        
        % Park-Transformation of the switchingstates factors
        Factors_d_q_x_y =single(zeros(4,1));
    
        Factors_d_q_x_y(3,1) = Factors_alpha_beta_x_y(3,Index);
        Factors_d_q_x_y(4,1) = Factors_alpha_beta_x_y(4,Index);
    
        Factors_d_q_x_y(1,1) = cos_theta_el*Factors_alpha_beta_x_y(1,Index)+sin_theta_el*Factors_alpha_beta_x_y(2,Index);
        Factors_d_q_x_y(2,1) = -sin_theta_el*Factors_alpha_beta_x_y(1,Index)+cos_theta_el*Factors_alpha_beta_x_y(2,Index);
    
        %Calculation of the voltages per switching state in alpha beta coordinates
        d_q_x_y_voltages_per_switching_state = single(u_dc_link_voltage*Factors_d_q_x_y);
    
        d_voltage_per_switching_state = d_q_x_y_voltages_per_switching_state(1,1);
        q_voltage_per_switching_state = d_q_x_y_voltages_per_switching_state(2,1);
        x_voltage_per_switching_state = d_q_x_y_voltages_per_switching_state(3,1);
        y_voltage_per_switching_state = d_q_x_y_voltages_per_switching_state(4,1);
    

end

== matlab function test_phase_voltages_without_delays/Phase_voltages_per_switching_state1/Subsystem/MATLAB Function3 ==
  data: sin_theta_el input; cos_theta_el input; d_voltage_per_switching_state output; u_dc_link_voltage input; Index input; q_voltage_per_switching_state output; x_voltage_per_switching_state output; y_voltage_per_switching_state output
function [d_voltage_per_switching_state, q_voltage_per_switching_state, x_voltage_per_switching_state, y_voltage_per_switching_state] = fcn(sin_theta_el, cos_theta_el, u_dc_link_voltage, Index)
      
        % Initial condition
            Index = Index+1;

    
        % Swichtingstates factors alpha beta x y
        Factors_alpha_beta_x_y = single([-0.288675134594813	 0.0446581987385205  -0.455341801261480	  -0.122008467928146;
                                         -0.166666666666667	-0.166666666666667	  0.122008467928146	   0.122008467928146;
                                         0.288675134594813	 0.622008467928146	  0.122008467928146	   0.455341801261480;
                                         -0.166666666666667	-0.166666666666667	 -0.455341801261480	  -0.455341801261480]);
        
        % Park-Transformation of the switchingstates factors
        Factors_d_q_x_y =single(zeros(4,1));
    
        Factors_d_q_x_y(3,1) = Factors_alpha_beta_x_y(3,Index);
        Factors_d_q_x_y(4,1) = Factors_alpha_beta_x_y(4,Index);
    
        Factors_d_q_x_y(1,1) = cos_theta_el*Factors_alpha_beta_x_y(1,Index)+sin_theta_el*Factors_alpha_beta_x_y(2,Index);
        Factors_d_q_x_y(2,1) = -sin_theta_el*Factors_alpha_beta_x_y(1,Index)+cos_theta_el*Factors_alpha_beta_x_y(2,Index);
    
        %Calculation of the voltages per switching state in alpha beta coordinates
        d_q_x_y_voltages_per_switching_state = single(u_dc_link_voltage*Factors_d_q_x_y);
    
        d_voltage_per_switching_state = d_q_x_y_voltages_per_switching_state(1,1);
        q_voltage_per_switching_state = d_q_x_y_voltages_per_switching_state(2,1);
        x_voltage_per_switching_state = d_q_x_y_voltages_per_switching_state(3,1);
        y_voltage_per_switching_state = d_q_x_y_voltages_per_switching_state(4,1);
    

end

== matlab function test_phase_voltages_without_delays/Phase_voltages_per_switching_state1/Subsystem/MATLAB Function4 ==
  data: sin_theta_el input; cos_theta_el input; d_voltage_per_switching_state output; u_dc_link_voltage input; Index input; q_voltage_per_switching_state output; x_voltage_per_switching_state output; y_voltage_per_switching_state output
function [d_voltage_per_switching_state, q_voltage_per_switching_state, x_voltage_per_switching_state, y_voltage_per_switching_state] = fcn(sin_theta_el, cos_theta_el, u_dc_link_voltage, Index)
      
        % Initial condition
            Index = Index+1;

    
        % Swichtingstates factors alpha beta x y
        Factors_alpha_beta_x_y = single([0.122008467928146	 0.455341801261480	-0.0446581987385205  0.288675134594813;
                                         -0.455341801261480	-0.455341801261480	-0.166666666666667	-0.166666666666667;
                                         -0.455341801261480	-0.122008467928146	-0.622008467928146	-0.288675134594813;
                                         0.122008467928146	 0.122008467928146	-0.166666666666667	-0.166666666666667]);
        
        % Park-Transformation of the switchingstates factors
        Factors_d_q_x_y =single(zeros(4,1));
    
        Factors_d_q_x_y(3,1) = Factors_alpha_beta_x_y(3,Index);
        Factors_d_q_x_y(4,1) = Factors_alpha_beta_x_y(4,Index);
   
        Factors_d_q_x_y(1,1) = cos_theta_el*Factors_alpha_beta_x_y(1,Index)+sin_theta_el*Factors_alpha_beta_x_y(2,Index);
        Factors_d_q_x_y(2,1) = -sin_theta_el*Factors_alpha_beta_x_y(1,Index)+cos_theta_el*Factors_alpha_beta_x_y(2,Index);
    
        %Calculation of the voltages per switching state in alpha beta coordinates
        d_q_x_y_voltages_per_switching_state = single(u_dc_link_voltage*Factors_d_q_x_y);
    
        d_voltage_per_switching_state = d_q_x_y_voltages_per_switching_state(1,1);
        q_voltage_per_switching_state = d_q_x_y_voltages_per_switching_state(2,1);
        x_voltage_per_switching_state = d_q_x_y_voltages_per_switching_state(3,1);
        y_voltage_per_switching_state = d_q_x_y_voltages_per_switching_state(4,1);
    

end

== matlab function test_phase_voltages_without_delays/Phase_voltages_per_switching_state1/MATLAB Function1 ==
  settings: fimath=fimath('RoundingMethod', 'Floor','OverflowAction', 'Wrap','ProductMode', 'FullPrecision', 'SumMode', 'FullPrecision')
  data: u input; y output
function y = fcn(u)

    y = u*(1/(2*pi));

end

== matlab function test_phase_voltages_without_delays/Phase_voltages_per_switching_state1/Subsystem/MATLAB Function5 ==
  data: sin_theta_el input; cos_theta_el input; d_voltage_per_switching_state output; u_dc_link_voltage input; Index input; q_voltage_per_switching_state output; x_voltage_per_switching_state output; y_voltage_per_switching_state output
function [d_voltage_per_switching_state, q_voltage_per_switching_state, x_voltage_per_switching_state, y_voltage_per_switching_state] = fcn(sin_theta_el, cos_theta_el, u_dc_link_voltage, Index)
      
        % Initial condition
            Index = Index+1;

    
        % Swichtingstates factors alpha beta x y
        Factors_alpha_beta_x_y = single([0.288675134594813	 0.622008467928146	 0.122008467928146	 0.455341801261480;
                                         -0.166666666666667	-0.166666666666667	 0.122008467928146	 0.122008467928146;
                                         -0.288675134594813	 0.0446581987385205	-0.455341801261480	-0.122008467928146;
                                         -0.166666666666667	-0.166666666666667	-0.455341801261480	-0.455341801261480]);
        
        % Park-Transformation of the switchingstates factors
        Factors_d_q_x_y =single(zeros(4,1));
    
        Factors_d_q_x_y(3,1) = Factors_alpha_beta_x_y(3,Index);
        Factors_d_q_x_y(4,1) = Factors_alpha_beta_x_y(4,Index);
    
        Factors_d_q_x_y(1,1) = cos_theta_el*Factors_alpha_beta_x_y(1,Index)+sin_theta_el*Factors_alpha_beta_x_y(2,Index);
        Factors_d_q_x_y(2,1) = -sin_theta_el*Factors_alpha_beta_x_y(1,Index)+cos_theta_el*Factors_alpha_beta_x_y(2,Index);
    
        %Calculation of the voltages per switching state in alpha beta coordinates
        d_q_x_y_voltages_per_switching_state = single(u_dc_link_voltage*Factors_d_q_x_y);
    
        d_voltage_per_switching_state = d_q_x_y_voltages_per_switching_state(1,1);
        q_voltage_per_switching_state = d_q_x_y_voltages_per_switching_state(2,1);
        x_voltage_per_switching_state = d_q_x_y_voltages_per_switching_state(3,1);
        y_voltage_per_switching_state = d_q_x_y_voltages_per_switching_state(4,1);
    

end

== matlab function test_phase_voltages_without_delays/Phase_voltages_per_switching_state1/Subsystem/MATLAB Function6 ==
  data: sin_theta_el input; cos_theta_el input; d_voltage_per_switching_state output; u_dc_link_voltage input; Index input; q_voltage_per_switching_state output; x_voltage_per_switching_state output; y_voltage_per_switching_state output
function [d_voltage_per_switching_state, q_voltage_per_switching_state, x_voltage_per_switching_state, y_voltage_per_switching_state] = fcn(sin_theta_el, cos_theta_el, u_dc_link_voltage, Index)
      
        % Initial condition
            Index = Index+1;

    
        % Swichtingstates factors alpha beta x y
        Factors_alpha_beta_x_y = single([-0.166666666666667	  0.166666666666667	    -0.333333333333333	 0;
                                         -0.622008467928146	 -0.622008467928146	    -0.333333333333333	-0.333333333333333;
                                         -0.166666666666667	  0.166666666666667	    -0.333333333333333	 0;
                                         -0.0446581987385205 -0.0446581987385205	-0.333333333333333	-0.333333333333333]);
        
        % Park-Transformation of the switchingstates factors
        Factors_d_q_x_y =single(zeros(4,1));
    
        Factors_d_q_x_y(3,1) = Factors_alpha_beta_x_y(3,Index);
        Factors_d_q_x_y(4,1) = Factors_alpha_beta_x_y(4,Index);
       
        Factors_d_q_x_y(1,1) = cos_theta_el*Factors_alpha_beta_x_y(1,Index)+sin_theta_el*Factors_alpha_beta_x_y(2,Index);
        Factors_d_q_x_y(2,1) = -sin_theta_el*Factors_alpha_beta_x_y(1,Index)+cos_theta_el*Factors_alpha_beta_x_y(2,Index);
    
        %Calculation of the voltages per switching state in alpha beta coordinates
        d_q_x_y_voltages_per_switching_state = single(u_dc_link_voltage*Factors_d_q_x_y);
    
        d_voltage_per_switching_state = d_q_x_y_voltages_per_switching_state(1,1);
        q_voltage_per_switching_state = d_q_x_y_voltages_per_switching_state(2,1);
        x_voltage_per_switching_state = d_q_x_y_voltages_per_switching_state(3,1);
        y_voltage_per_switching_state = d_q_x_y_voltages_per_switching_state(4,1);
    

end

== matlab function test_phase_voltages_without_delays/Phase_voltages_per_switching_state1/Subsystem/MATLAB Function7 ==
  data: sin_theta_el input; cos_theta_el input; d_voltage_per_switching_state output; u_dc_link_voltage input; Index input; q_voltage_per_switching_state output; x_voltage_per_switching_state output; y_voltage_per_switching_state output
function [d_voltage_per_switching_state, q_voltage_per_switching_state, x_voltage_per_switching_state, y_voltage_per_switching_state] = fcn(sin_theta_el, cos_theta_el, u_dc_link_voltage, Index)
      
        % Initial condition
            Index = Index+1;

    
        % Swichtingstates factors alpha beta x y
        Factors_alpha_beta_x_y = single([0	                 0.333333333333333	-0.166666666666667	  0.166666666666667;
                                         -0.333333333333333	-0.333333333333333	-0.0446581987385205	 -0.0446581987385205;
                                         0	                 0.333333333333333	-0.166666666666667	  0.166666666666667;
                                         -0.333333333333333	-0.333333333333333	-0.622008467928146	 -0.622008467928146]);
        
        % Park-Transformation of the switchingstates factors
        Factors_d_q_x_y =single(zeros(4,1));
    
        Factors_d_q_x_y(3,1) = Factors_alpha_beta_x_y(3,Index);
        Factors_d_q_x_y(4,1) = Factors_alpha_beta_x_y(4,Index);
    
        Factors_d_q_x_y(1,1) = cos_theta_el*Factors_alpha_beta_x_y(1,Index)+sin_theta_el*Factors_alpha_beta_x_y(2,Index);
        Factors_d_q_x_y(2,1) = -sin_theta_el*Factors_alpha_beta_x_y(1,Index)+cos_theta_el*Factors_alpha_beta_x_y(2,Index);
    
        %Calculation of the voltages per switching state in alpha beta coordinates
        d_q_x_y_voltages_per_switching_state = single(u_dc_link_voltage*Factors_d_q_x_y);
    
        d_voltage_per_switching_state = d_q_x_y_voltages_per_switching_state(1,1);
        q_voltage_per_switching_state = d_q_x_y_voltages_per_switching_state(2,1);
        x_voltage_per_switching_state = d_q_x_y_voltages_per_switching_state(3,1);
        y_voltage_per_switching_state = d_q_x_y_voltages_per_switching_state(4,1);
    

end

== matlab function test_phase_voltages_without_delays/Phase_voltages_per_switching_state1/Subsystem/MATLAB Function8 ==
  data: sin_theta_el input; cos_theta_el input; d_voltage_per_switching_state output; u_dc_link_voltage input; Index input; q_voltage_per_switching_state output; x_voltage_per_switching_state output; y_voltage_per_switching_state output
function [d_voltage_per_switching_state, q_voltage_per_switching_state, x_voltage_per_switching_state, y_voltage_per_switching_state] = fcn(sin_theta_el, cos_theta_el, u_dc_link_voltage, Index)
      
        % Initial condition
            Index = Index+1;

    
        % Swichtingstates factors alpha beta x y
        Factors_alpha_beta_x_y = single([-0.166666666666667	 0.166666666666667	 -0.333333333333333	0;
                                         0.0446581987385205	 0.0446581987385205	  0.333333333333333	0.333333333333333;
                                         -0.166666666666667	 0.166666666666667	 -0.333333333333333	0;
                                         0.622008467928146	 0.622008467928146	  0.333333333333333	0.333333333333333]);
        
        % Park-Transformation of the switchingstates factors
        Factors_d_q_x_y =single(zeros(4,1));
    
        Factors_d_q_x_y(3,1) = Factors_alpha_beta_x_y(3,Index);
        Factors_d_q_x_y(4,1) = Factors_alpha_beta_x_y(4,Index);
       
        Factors_d_q_x_y(1,1) = cos_theta_el*Factors_alpha_beta_x_y(1,Index)+sin_theta_el*Factors_alpha_beta_x_y(2,Index);
        Factors_d_q_x_y(2,1) = -sin_theta_el*Factors_alpha_beta_x_y(1,Index)+cos_theta_el*Factors_alpha_beta_x_y(2,Index);
    
        %Calculation of the voltages per switching state in alpha beta coordinates
        d_q_x_y_voltages_per_switching_state = single(u_dc_link_voltage*Factors_d_q_x_y);
    
        d_voltage_per_switching_state = d_q_x_y_voltages_per_switching_state(1,1);
        q_voltage_per_switching_state = d_q_x_y_voltages_per_switching_state(2,1);
        x_voltage_per_switching_state = d_q_x_y_voltages_per_switching_state(3,1);
        y_voltage_per_switching_state = d_q_x_y_voltages_per_switching_state(4,1);
    

end

== matlab function test_phase_voltages_without_delays/Phase_voltages_per_switching_state1/Subsystem/MATLAB Function9 ==
  data: sin_theta_el input; cos_theta_el input; d_voltage_per_switching_state output; u_dc_link_voltage input; Index input; q_voltage_per_switching_state output; x_voltage_per_switching_state output; y_voltage_per_switching_state output
function [d_voltage_per_switching_state, q_voltage_per_switching_state, x_voltage_per_switching_state, y_voltage_per_switching_state] = fcn(sin_theta_el, cos_theta_el, u_dc_link_voltage, Index)
      
        % Initial condition
            Index = Index+1;

    
        % Swichtingstates factors alpha beta x y
        Factors_alpha_beta_x_y = single([0	                0.333333333333333	-0.166666666666667  	0.166666666666667;
                                         0.333333333333333	0.333333333333333	 0.622008467928146	    0.622008467928146;
                                         0	                0.333333333333333	-0.166666666666667	    0.166666666666667;
                                         0.333333333333333	0.333333333333333	 0.0446581987385205 	0.0446581987385205]);
        
        % Park-Transformation of the switchingstates factors
        Factors_d_q_x_y =single(zeros(4,1));
    
        Factors_d_q_x_y(3,1) = Factors_alpha_beta_x_y(3,Index);
        Factors_d_q_x_y(4,1) = Factors_alpha_beta_x_y(4,Index);
       
        Factors_d_q_x_y(1,1) = cos_theta_el*Factors_alpha_beta_x_y(1,Index)+sin_theta_el*Factors_alpha_beta_x_y(2,Index);
        Factors_d_q_x_y(2,1) = -sin_theta_el*Factors_alpha_beta_x_y(1,Index)+cos_theta_el*Factors_alpha_beta_x_y(2,Index);
    
        %Calculation of the voltages per switching state in alpha beta coordinates
        d_q_x_y_voltages_per_switching_state = single(u_dc_link_voltage*Factors_d_q_x_y);
    
        d_voltage_per_switching_state = d_q_x_y_voltages_per_switching_state(1,1);
        q_voltage_per_switching_state = d_q_x_y_voltages_per_switching_state(2,1);
        x_voltage_per_switching_state = d_q_x_y_voltages_per_switching_state(3,1);
        y_voltage_per_switching_state = d_q_x_y_voltages_per_switching_state(4,1);
    

end

== matlab function test_phase_voltages_without_delays/Phase_voltages_per_switching_state1/Subsystem/MATLAB Function ==
  data: sin_theta_el input; cos_theta_el input; d_voltage_per_switching_state output; u_dc_link_voltage input; Index input; q_voltage_per_switching_state output; x_voltage_per_switching_state output; y_voltage_per_switching_state output
function [d_voltage_per_switching_state, q_voltage_per_switching_state, x_voltage_per_switching_state, y_voltage_per_switching_state] = fcn(sin_theta_el, cos_theta_el, u_dc_link_voltage, Index)
      
        % Initial condition
            Index = Index+1;

    
        % Swichtingstates factors alpha beta x y
        Factors_alpha_beta_x_y = single([-0.166666666666667	 0.166666666666667	-0.333333333333333	0;
                                         -0.288675134594813	-0.288675134594813	 0	                0;
                                         -0.166666666666667	 0.166666666666667	-0.333333333333333	0;
                                         0.288675134594813	 0.288675134594813	 0	                0]);
        
        % Park-Transformation of the switchingstates factors
        Factors_d_q_x_y =single(zeros(4,1));
    
        Factors_d_q_x_y(3,1) = Factors_alpha_beta_x_y(3,Index);
        Factors_d_q_x_y(4,1) = Factors_alpha_beta_x_y(4,Index);

        Factors_d_q_x_y(1,1) = cos_theta_el*Factors_alpha_beta_x_y(1,Index)+sin_theta_el*Factors_alpha_beta_x_y(2,Index);
        Factors_d_q_x_y(2,1) = -sin_theta_el*Factors_alpha_beta_x_y(1,Index)+cos_theta_el*Factors_alpha_beta_x_y(2,Index);
    
        %Calculation of the voltages per switching state in alpha beta coordinates
        d_q_x_y_voltages_per_switching_state = single(u_dc_link_voltage*Factors_d_q_x_y);
    
        d_voltage_per_switching_state = d_q_x_y_voltages_per_switching_state(1,1);
        q_voltage_per_switching_state = d_q_x_y_voltages_per_switching_state(2,1);
        x_voltage_per_switching_state = d_q_x_y_voltages_per_switching_state(3,1);
        y_voltage_per_switching_state = d_q_x_y_voltages_per_switching_state(4,1);
    

end
